simulink model "encoder_teta"  (R2017b)
settings: Solver=VariableStepAuto  StartTime=0.0  StopTime=10.0  RelTol=1e-3
settings Model: Creator=ACER  LastModifiedBy=ACER

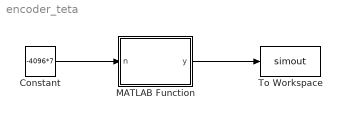
== system encoder_teta ==
  Constant : Constant  Value=-4096*7
  MATLAB Function : MATLAB Function  TreatAsAtomicUnit=on
  To Workspace : ToWorkspace  VariableName=simout  SampleTime=-1
  wires:
  Constant/1 -> MATLAB Function/1(n)
  MATLAB Function/1(y) -> To Workspace/1

== matlab function encoder_teta/MATLAB Function ==
  data: n input; y output
function y = fcn(n)
if(n>=0)
  floor1=floor(n/8192);
  if(rem(floor1, 2)==0)
      n0=180;
      deg=(n-floor1*8192)*180/(2*4096);
      y = n0-deg;
  else
      deg=(n-floor1*8192)*180/(2*4096);
      y = -1*deg;
  end 
else
    floor1=floor(n/8192);
    floor1=floor1+1;
    if(rem(floor1, 2)==0)
        n0=180;
        deg=(n-floor1*8192)*180/(2*4096);
        y = -1*(n0+deg);
    else
        deg=(n-floor1*8192)*180/(2*4096);
        y = -1*deg;
    end
end
